simulink model "FCS_MPC_6ph_testbench"  (R2022a)
settings: Solver=ode23t  StartTime=0.0  StopTime=0.1  RelTol=1e-3  AbsTol=1e-3  EnableMultiTasking=on
values from neighbouring files (symbols this model uses):
  f_c = 100000    [Params_testbench.m]
  L_d = 0.0001473    [Params_testbench.m]
  L_q = 0.0001484    [Params_testbench.m]
  L_x = 0.00005566    (= 5.566e-05)    [Params_testbench.m]
  L_y = L_x    (= 5.566e-05)    [Params_testbench.m]
  p = 5    [Params_testbench.m]
  psi_pm = 0.0048    [Params_testbench.m]
  R_ph = 0.1278    [Params_testbench.m]
  u_dc = 36.0    (= 36)    [Params_testbench.m]
libraries: nesl_utility x39, fl_lib x32, hdlsllib x25, ee_lib x12, simulink x2, spsAlphaBetaZerotodq0Lib x1
(part 3 of 4)

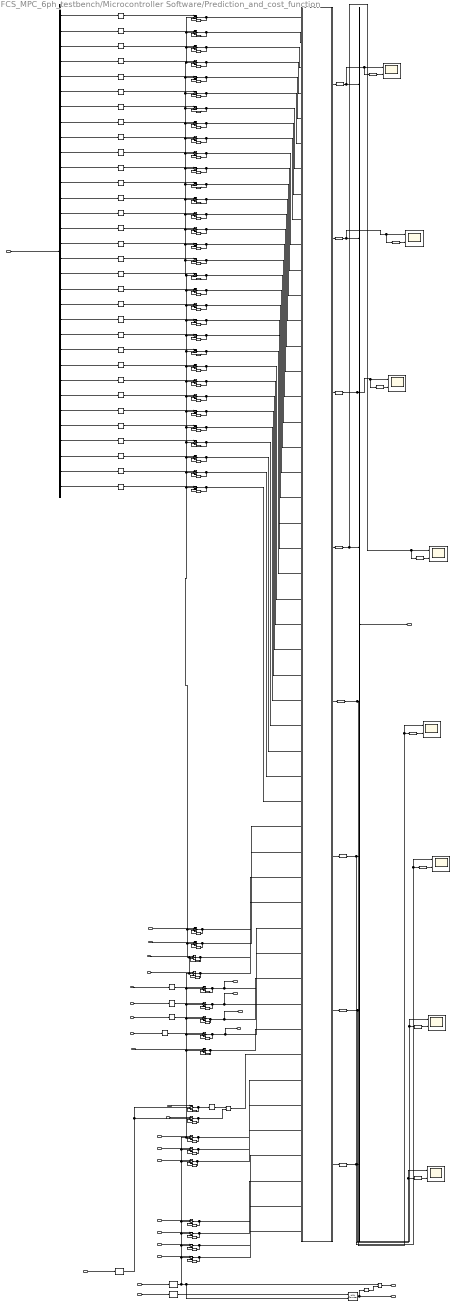
== system FCS_MPC_6ph_testbench/Microcontroller Software/Prediction_and_cost_function ==
  Lq_AXI : Inport
  Ld_AXI : Inport  Port=2
  SampleTime_div_Ld_AXI : Inport  Port=3
  SampleTime_div_Lq_AXI : Inport  Port=4
  SampleTime_div_Lx_AXI : Inport  Port=5
  SampleTime_div_Ly_AXI : Inport  Port=6
  id_k_1 : Inport  Port=7
  iq_k_1 : Inport  Port=8
  ix_k_1 : Inport  Port=9
  iy_k_1 : Inport  Port=10
  Rs_AXI : Inport  Port=11
  omega_m_measured : Inport  Port=12
  pole_pairs_AXI : Inport  Port=13
  psiPM_AXI : Inport  Port=14
  id_ref_AXI : Inport  Port=15
  iq_ref_AXI : Inport  Port=16
  ix_ref_AXI : Inport  Port=17
  iy_ref_AXI : Inport  Port=18
  valid_in : Inport  Port=19
  Reset : Inport  Port=20
  valid_in_ADC : Inport  Port=21
  dqxy_phase_voltage_per_switching_state : Inport  Port=22
  Compare To Constant : hdlsllib/Logic and Bit Operations/Compare To Constant  relop=<=  const=8  OutDataTypeStr=boolean
      settings: SourceProductBaseCode=SL
  Data Type Conversion{1..17,19..38} (37 alike) : DataTypeConversion  OutDataTypeStr=single  RndMeth=Nearest  SaturateOnIntegerOverflow=off
  Data Type Conversion{18,39..52,54} (16 alike) : DataTypeConversion  OutDataTypeStr=fixdt(1,20,9)  SaturateOnIntegerOverflow=off  RndMeth=Floor
  Delay{1..4,8..20,33,104..135} (50 alike) : Delay  DelayLength=1
  Demux : Demux  Outputs=32
  Detect Rise Positive : hdlsllib/Logic and Bit Operations/Detect Rise Positive  vinit=0  OutDataTypeStr=boolean
      settings: SourceProductBaseCode=SL
  Detect Rise Positive1 : hdlsllib/Logic and Bit Operations/Detect Rise Positive  vinit=0  OutDataTypeStr=boolean
      settings: SourceProductBaseCode=SL
  Detect Rise Positive2 : hdlsllib/Logic and Bit Operations/Detect Rise Positive  vinit=0  OutDataTypeStr=boolean
      settings: SourceProductBaseCode=SL
  HDL Counter : hdlsllib/Sources/HDL Counter  CountType=Free running  CountInit=0  CountStep=1  CountMax=25  CountFromType=Initial value  CountFrom=0  CountResetPort=on  CountLoadPort=off  CountEnbPort=on  CountDirPort=off  CountHitOutputPort=off  CountDataType=Signed  CountWordLen=32  CountFracLen=0  CountSampTime=1
  J_fixed_point{,1..7} (8 alike) : Scope  NumInputPorts=2
  Logical Operator : Logic  AllPortsSameDT=off  OutDataTypeStr=boolean
  Mux : Mux  Inputs=8
  Product : Product  Inputs=**
  Subsystem : Subsystem
  Switch_on{1..4,8..10,12..21,59..90} (49 alike) : Switch  Threshold=1  OutDataTypeStr=single  RndMeth=Simplest  SaturateOnIntegerOverflow=off  InputSameDT=off
  Switch_on11 : Switch  Threshold=1  RndMeth=Simplest  SaturateOnIntegerOverflow=off  InputSameDT=off  OutDataTypeStr=Inherit: Same as first input
  done : Outport
  Index : Outport  Port=2
  J : Outport  Port=3
  id_k_1_Prediction : Outport  Port=4
  iq_k_1_Prediction : Outport  Port=5
  ix_k_1_Prediction : Outport  Port=6
  iy_k_1_Prediction : Outport  Port=7
  wires:
  Switch_on12/1 -> Subsystem/41(Rs15), Delay12/1
  Rs_AXI/1 -> Switch_on12/1
  SampleTime_div_Ld_AXI/1 -> Switch_on21/1
  Delay3/1 -> Switch_on3/3
  Delay10/1 -> Switch_on10/3
  iq_ref_AXI/1 -> Switch_on2/1
  Delay17/1 -> Switch_on18/3
  Switch_on10/1 -> Delay10/1, Subsystem/43(Lq15)
  Delay11/1 -> Switch_on11/3
  SampleTime_div_Lq_AXI/1 -> Switch_on20/1
  Ld_AXI/1 -> Switch_on9/1
  psiPM_AXI/1 -> Switch_on8/1
  Delay1/1 -> Switch_on1/3
  id_ref_AXI/1 -> Switch_on3/1
  Product/1 -> Subsystem/42(omega_el15)  "omega_el"
  Delay9/1 -> Switch_on9/3
  Delay20/1 -> Switch_on21/3
  pole_pairs_AXI/1 -> Switch_on4/1
  Switch_on18/1 -> Delay17/1, Subsystem/36(SampleTime_div_Ly15)
  Delay19/1 -> Switch_on20/3
  Delay13/1 -> Switch_on13/3
  Switch_on15/1 -> Delay14/1, ix_k_1_Prediction/1, Subsystem/39(ix_k_16)
  Delay18/1 -> Switch_on19/3
  Switch_on19/1 -> Delay18/1, Subsystem/35(SampleTime_div_Lx15)
  Switch_on20/1 -> Delay19/1, Subsystem/34(SampleTime_div_Lq15)
  Switch_on13/1 -> Delay13/1, iy_k_1_Prediction/1, Subsystem/40(iy_k_16)
  iy_ref_AXI/1 -> Switch_on14/1
  Delay2/1 -> Switch_on2/3
  Delay16/1 -> Switch_on17/3
  Switch_on17/1 -> Delay16/1, id_k_1_Prediction/1, Subsystem/37(id_k_16)
  Delay15/1 -> Switch_on16/3
  Switch_on16/1 -> Delay15/1, iq_k_1_Prediction/1, Subsystem/38(iq_k_16)
  Switch_on11/1 -> Data Type Conversion4/1, Delay11/1
  Delay33/1 -> Switch_on14/3
  SampleTime_div_Lx_AXI/1 -> Switch_on19/1
  Switch_on14/1 -> Delay33/1, Subsystem/49(iy_ref15)
  Delay12/1 -> Switch_on12/3
  valid_in/1 -> Detect Rise Positive/1
  Switch_on3/1 -> Delay3/1, Subsystem/46(id_ref15)
  Switch_on21/1 -> Delay20/1, Subsystem/33(SampleTime_div_Ld15)
  Switch_on2/1 -> Delay2/1, Subsystem/47(iq_ref15)
  Lq_AXI/1 -> Switch_on10/1
  Switch_on1/1 -> Delay1/1, Subsystem/48(ix_ref15)
  Switch_on9/1 -> Delay9/1, Subsystem/44(Ld15)
  SampleTime_div_Ly_AXI/1 -> Switch_on18/1
  Delay14/1 -> Switch_on15/3
  ix_ref_AXI/1 -> Switch_on1/1
  Switch_on8/1 -> Delay8/1, Subsystem/45(psiPM15)
  Delay8/1 -> Switch_on8/3
  id_k_1/1 -> Data Type Conversion7/1
  iq_k_1/1 -> Data Type Conversion8/1
  ix_k_1/1 -> Data Type Conversion9/1
  iy_k_1/1 -> Data Type Conversion10/1
  omega_m_measured/1 -> Switch_on11/1
  Reset/1 -> Detect Rise Positive1/1
  Detect Rise Positive1/1 -> HDL Counter/1  "End_Cycle"
  Compare To Constant/1 -> Logical Operator/2
  HDL Counter/1 -> Index/1, Compare To Constant/1
  valid_in_ADC/1 -> Detect Rise Positive2/1
  Mux/1 -> J/1
  Switch_on61/1 -> Subsystem/30(q_phase_voltage_per_switching_state7), Delay106/1
  Delay106/1 -> Switch_on61/3
  Delay107/1 -> Switch_on62/3
  Switch_on62/1 -> Subsystem/29(d_phase_voltage_per_switching_state7), Delay107/1
  Delay104/1 -> Switch_on59/3
  Switch_on59/1 -> Subsystem/32(y_phase_voltage_per_switching_state7), Delay104/1
  Delay105/1 -> Switch_on60/3
  Switch_on60/1 -> Subsystem/31(x_phase_voltage_per_switching_state7), Delay105/1
  Switch_on65/1 -> Subsystem/26(q_phase_voltage_per_switching_state6), Delay110/1
  Delay110/1 -> Switch_on65/3
  Delay111/1 -> Switch_on66/3
  Switch_on66/1 -> Subsystem/25(d_phase_voltage_per_switching_state6), Delay111/1
  Delay108/1 -> Switch_on63/3
  Switch_on63/1 -> Subsystem/28(y_phase_voltage_per_switching_state6), Delay108/1
  Delay109/1 -> Switch_on64/3
  Switch_on64/1 -> Subsystem/27(x_phase_voltage_per_switching_state6), Delay109/1
  Switch_on69/1 -> Subsystem/22(q_phase_voltage_per_switching_state5), Delay114/1
  Delay114/1 -> Switch_on69/3
  Delay115/1 -> Switch_on70/3
  Switch_on70/1 -> Subsystem/21(d_phase_voltage_per_switching_state5), Delay115/1
  Delay112/1 -> Switch_on67/3
  Switch_on67/1 -> Subsystem/24(y_phase_voltage_per_switching_state5), Delay112/1
  Delay113/1 -> Switch_on68/3
  Switch_on68/1 -> Subsystem/23(x_phase_voltage_per_switching_state5), Delay113/1
  Switch_on73/1 -> Subsystem/18(q_phase_voltage_per_switching_state4), Delay118/1
  Delay118/1 -> Switch_on73/3
  Delay119/1 -> Switch_on74/3
  Switch_on74/1 -> Subsystem/17(d_phase_voltage_per_switching_state4), Delay119/1
  Delay116/1 -> Switch_on71/3
  Switch_on71/1 -> Subsystem/20(y_phase_voltage_per_switching_state4), Delay116/1
  Delay117/1 -> Switch_on72/3
  Switch_on72/1 -> Subsystem/19(x_phase_voltage_per_switching_state4), Delay117/1
  Switch_on77/1 -> Subsystem/14(q_phase_voltage_per_switching_state3), Delay122/1
  Delay122/1 -> Switch_on77/3
  Delay123/1 -> Switch_on78/3
  Switch_on78/1 -> Subsystem/13(d_phase_voltage_per_switching_state3), Delay123/1
  Delay120/1 -> Switch_on75/3
  Switch_on75/1 -> Subsystem/16(y_phase_voltage_per_switching_state3), Delay120/1
  Delay121/1 -> Switch_on76/3
  Switch_on76/1 -> Subsystem/15(x_phase_voltage_per_switching_state3), Delay121/1
  Switch_on81/1 -> Subsystem/10(q_phase_voltage_per_switching_state2), Delay126/1
  Delay126/1 -> Switch_on81/3
  Delay127/1 -> Switch_on82/3
  Switch_on82/1 -> Subsystem/9(d_phase_voltage_per_switching_state2), Delay127/1
  Delay124/1 -> Switch_on79/3
  Switch_on79/1 -> Subsystem/12(y_phase_voltage_per_switching_state2), Delay124/1
  Delay125/1 -> Switch_on80/3
  Switch_on80/1 -> Subsystem/11(x_phase_voltage_per_switching_state2), Delay125/1
  Switch_on85/1 -> Subsystem/6(q_phase_voltage_per_switching_state1), Delay130/1
  Delay130/1 -> Switch_on85/3
  Delay131/1 -> Switch_on86/3
  Switch_on86/1 -> Subsystem/5(d_phase_voltage_per_switching_state1), Delay131/1
  Delay128/1 -> Switch_on83/3
  Switch_on83/1 -> Subsystem/8(y_phase_voltage_per_switching_state1), Delay128/1
  Delay129/1 -> Switch_on84/3
  Switch_on84/1 -> Subsystem/7(x_phase_voltage_per_switching_state1), Delay129/1
  Switch_on89/1 -> Subsystem/2(q_phase_voltage_per_switching_state), Delay134/1
  Delay134/1 -> Switch_on89/3
  Delay135/1 -> Switch_on90/3
  Switch_on90/1 -> Subsystem/1(d_phase_voltage_per_switching_state), Delay135/1
  Delay132/1 -> Switch_on87/3
  Switch_on87/1 -> Subsystem/4(y_phase_voltage_per_switching_state), Delay132/1
  Delay133/1 -> Switch_on88/3
  Switch_on88/1 -> Subsystem/3(x_phase_voltage_per_switching_state), Delay133/1
  Detect Rise Positive/1 -> Logical Operator/1, HDL Counter/2, Switch_on14/2, Switch_on1/2, Switch_on8/2, Switch_on9/2, Switch_on12/2, Switch_on20/2, Switch_on90/2, Switch_on89/2, Switch_on88/2, Switch_on87/2, Switch_on86/2, Switch_on85/2, Switch_on84/2, Switch_on83/2, Switch_on82/2, Switch_on81/2, Switch_on80/2, Switch_on79/2, Switch_on78/2, Switch_on77/2, Switch_on76/2, Switch_on75/2, Switch_on74/2, Switch_on73/2, Switch_on72/2, Switch_on71/2, Switch_on70/2, Switch_on69/2, Switch_on68/2, Switch_on67/2, Switch_on66/2, Switch_on65/2, Switch_on64/2, Switch_on63/2, Switch_on62/2, Switch_on61/2, Switch_on60/2, Switch_on59/2, Switch_on21/2, Switch_on19/2, Switch_on18/2, Switch_on17/2, Switch_on16/2, Switch_on15/2, Switch_on13/2, Switch_on10/2, Switch_on3/2, Switch_on2/2  "End_Cycle"
  Demux/32 -> Data Type Conversion38/1
  Demux/31 -> Data Type Conversion37/1
  Demux/30 -> Data Type Conversion36/1
  Demux/29 -> Data Type Conversion35/1
  Demux/28 -> Data Type Conversion34/1
  Demux/27 -> Data Type Conversion33/1
  Demux/26 -> Data Type Conversion32/1
  Demux/25 -> Data Type Conversion31/1
  Demux/24 -> Data Type Conversion30/1
  Demux/23 -> Data Type Conversion29/1
  Demux/22 -> Data Type Conversion28/1
  Demux/21 -> Data Type Conversion27/1
  Demux/20 -> Data Type Conversion26/1
  Demux/19 -> Data Type Conversion25/1
  Demux/18 -> Data Type Conversion24/1
  Demux/17 -> Data Type Conversion23/1
  Demux/16 -> Data Type Conversion22/1
  Demux/15 -> Data Type Conversion21/1
  Demux/14 -> Data Type Conversion20/1
  Demux/13 -> Data Type Conversion19/1
  Demux/12 -> Data Type Conversion17/1
  Demux/11 -> Data Type Conversion16/1
  Demux/10 -> Data Type Conversion15/1
  Demux/9 -> Data Type Conversion14/1
  Demux/8 -> Data Type Conversion13/1
  Demux/7 -> Data Type Conversion12/1
  Demux/6 -> Data Type Conversion11/1
  Demux/5 -> Data Type Conversion6/1
  Demux/4 -> Data Type Conversion5/1
  Demux/3 -> Data Type Conversion3/1
  Demux/2 -> Data Type Conversion2/1
  Demux/1 -> Data Type Conversion1/1
  Logical Operator/1 -> done/1
  dqxy_phase_voltage_per_switching_state/1 -> Demux/1
  Data Type Conversion10/1 -> Switch_on13/1
  Data Type Conversion9/1 -> Switch_on15/1
  Data Type Conversion8/1 -> Switch_on16/1
  Data Type Conversion7/1 -> Switch_on17/1
  Data Type Conversion4/1 -> Product/1
  Data Type Conversion38/1 -> Switch_on59/1
  Data Type Conversion37/1 -> Switch_on60/1
  Data Type Conversion36/1 -> Switch_on61/1
  Data Type Conversion35/1 -> Switch_on62/1
  Data Type Conversion34/1 -> Switch_on63/1
  Data Type Conversion33/1 -> Switch_on64/1
  Data Type Conversion32/1 -> Switch_on65/1
  Data Type Conversion31/1 -> Switch_on66/1
  Data Type Conversion30/1 -> Switch_on67/1
  Data Type Conversion29/1 -> Switch_on68/1
  Data Type Conversion28/1 -> Switch_on69/1
  Data Type Conversion27/1 -> Switch_on70/1
  Data Type Conversion26/1 -> Switch_on71/1
  Data Type Conversion25/1 -> Switch_on72/1
  Data Type Conversion24/1 -> Switch_on73/1
  Data Type Conversion23/1 -> Switch_on74/1
  Data Type Conversion22/1 -> Switch_on75/1
  Data Type Conversion21/1 -> Switch_on76/1
  Data Type Conversion20/1 -> Switch_on77/1
  Data Type Conversion19/1 -> Switch_on78/1
  Data Type Conversion17/1 -> Switch_on79/1
  Data Type Conversion16/1 -> Switch_on80/1
  Data Type Conversion15/1 -> Switch_on81/1
  Data Type Conversion14/1 -> Switch_on82/1
  Data Type Conversion13/1 -> Switch_on83/1
  Data Type Conversion12/1 -> Switch_on84/1
  Data Type Conversion11/1 -> Switch_on85/1
  Data Type Conversion6/1 -> Switch_on86/1
  Data Type Conversion5/1 -> Switch_on87/1
  Data Type Conversion3/1 -> Switch_on88/1
  Data Type Conversion2/1 -> Switch_on89/1
  Data Type Conversion1/1 -> Switch_on90/1
  Detect Rise Positive2/1 -> Switch_on4/2, Switch_on11/2  "End_Cycle"
  Switch_on4/1 -> Product/2, Delay4/1
  Delay4/1 -> Switch_on4/3
  Data Type Conversion18/1 -> J_fixed_point/2  "fc"
  Data Type Conversion39/1 -> J_fixed_point1/2  "fc"
  Data Type Conversion40/1 -> J_fixed_point2/2  "fc"
  Data Type Conversion41/1 -> J_fixed_point3/2  "fc"
  Data Type Conversion42/1 -> J_fixed_point4/2  "fc"
  Data Type Conversion43/1 -> J_fixed_point5/2  "fc"
  Data Type Conversion44/1 -> J_fixed_point6/2  "fc"
  Data Type Conversion45/1 -> J_fixed_point7/2  "fc"
  Subsystem/8(J7) -> Data Type Conversion52/1  "fc"
  Subsystem/7(J6) -> Data Type Conversion51/1  "fc"
  Subsystem/6(J5) -> Data Type Conversion50/1  "fc"
  Subsystem/5(J4) -> Data Type Conversion49/1  "fc"
  Subsystem/4(J3) -> Data Type Conversion48/1  "fc"
  Subsystem/3(J2) -> Data Type Conversion47/1  "fc"
  Subsystem/2(J1) -> Data Type Conversion46/1  "fc"
  Subsystem/1(J) -> Data Type Conversion54/1  "fc"
  Data Type Conversion54/1 -> Data Type Conversion18/1, J_fixed_point/1, Mux/1  "fc"
  Data Type Conversion46/1 -> Data Type Conversion39/1, J_fixed_point1/1, Mux/2  "fc"
  Data Type Conversion47/1 -> Data Type Conversion40/1, J_fixed_point2/1, Mux/3  "fc"
  Data Type Conversion48/1 -> Data Type Conversion41/1, J_fixed_point3/1, Mux/4  "fc"
  Data Type Conversion49/1 -> J_fixed_point4/1, Data Type Conversion42/1, Mux/5  "fc"
  Data Type Conversion50/1 -> J_fixed_point5/1, Data Type Conversion43/1, Mux/6  "fc"
  Data Type Conversion51/1 -> J_fixed_point6/1, Data Type Conversion44/1, Mux/7  "fc"
  Data Type Conversion52/1 -> J_fixed_point7/1, Data Type Conversion45/1, Mux/8  "fc"

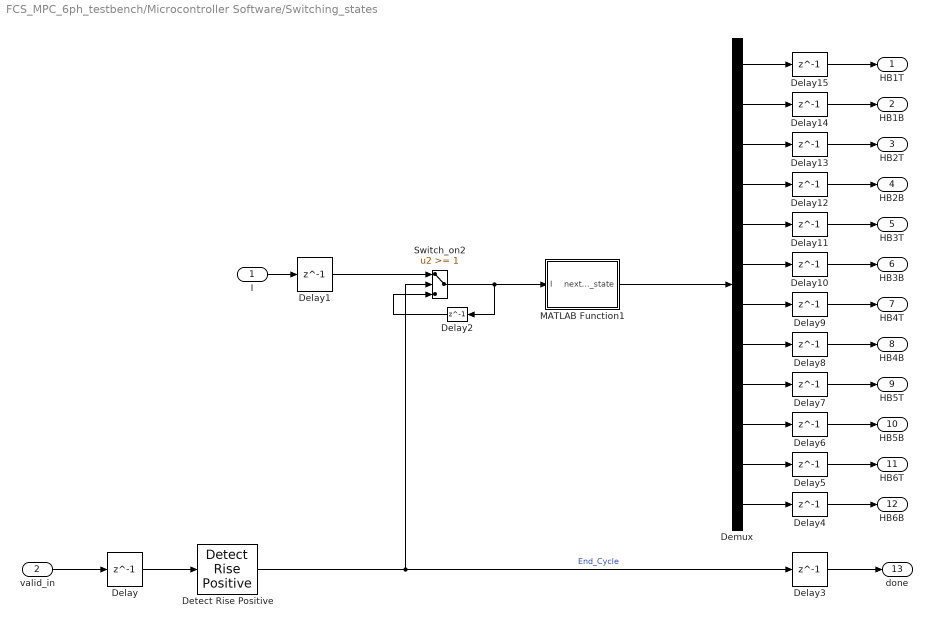
== system FCS_MPC_6ph_testbench/Microcontroller Software/Switching_states ==
  I : Inport
  valid_in : Inport  Port=2
  Delay{,1..15} (16 alike) : Delay  DelayLength=1
  Demux : Demux  Outputs=12
  Detect Rise Positive : hdlsllib/Logic and Bit Operations/Detect Rise Positive  vinit=0  OutDataTypeStr=boolean
      settings: SourceProductBaseCode=SL
  MATLAB Function1 : MATLAB Function  TreatAsAtomicUnit=on
  Switch_on2 : Switch  Threshold=1  OutDataTypeStr=Inherit: Inherit via back propagation  RndMeth=Simplest  SaturateOnIntegerOverflow=off  InputSameDT=off
  HB1T : Outport
  HB1B : Outport  Port=2
  HB2T : Outport  Port=3
  HB2B : Outport  Port=4
  HB3T : Outport  Port=5
  HB3B : Outport  Port=6
  HB4T : Outport  Port=7
  HB4B : Outport  Port=8
  HB5T : Outport  Port=9
  HB5B : Outport  Port=10
  HB6T : Outport  Port=11
  HB6B : Outport  Port=12
  done : Outport  Port=13
  wires:
  Demux/4 -> Delay12/1
  I/1 -> Delay1/1
  Demux/6 -> Delay10/1
  Demux/12 -> Delay4/1
  Demux/8 -> Delay8/1
  valid_in/1 -> Delay/1
  Demux/7 -> Delay9/1
  Demux/2 -> Delay14/1
  Detect Rise Positive/1 -> Delay3/1, Switch_on2/2  "End_Cycle"
  Demux/5 -> Delay11/1
  Delay2/1 -> Switch_on2/3
  Demux/1 -> Delay15/1
  Demux/9 -> Delay7/1
  Demux/10 -> Delay6/1
  MATLAB Function1/1(next_switching_state) -> Demux/1
  Demux/3 -> Delay13/1
  Delay/1 -> Detect Rise Positive/1
  Delay1/1 -> Switch_on2/1
  Delay3/1 -> done/1
  Delay4/1 -> HB6B/1
  Demux/11 -> Delay5/1
  Delay5/1 -> HB6T/1
  Delay6/1 -> HB5B/1
  Delay7/1 -> HB5T/1
  Delay8/1 -> HB4B/1
  Delay9/1 -> HB4T/1
  Delay10/1 -> HB3B/1
  Delay11/1 -> HB3T/1
  Delay12/1 -> HB2B/1
  Delay13/1 -> HB2T/1
  Delay14/1 -> HB1B/1
  Delay15/1 -> HB1T/1
  Switch_on2/1 -> MATLAB Function1/1(I), Delay2/1

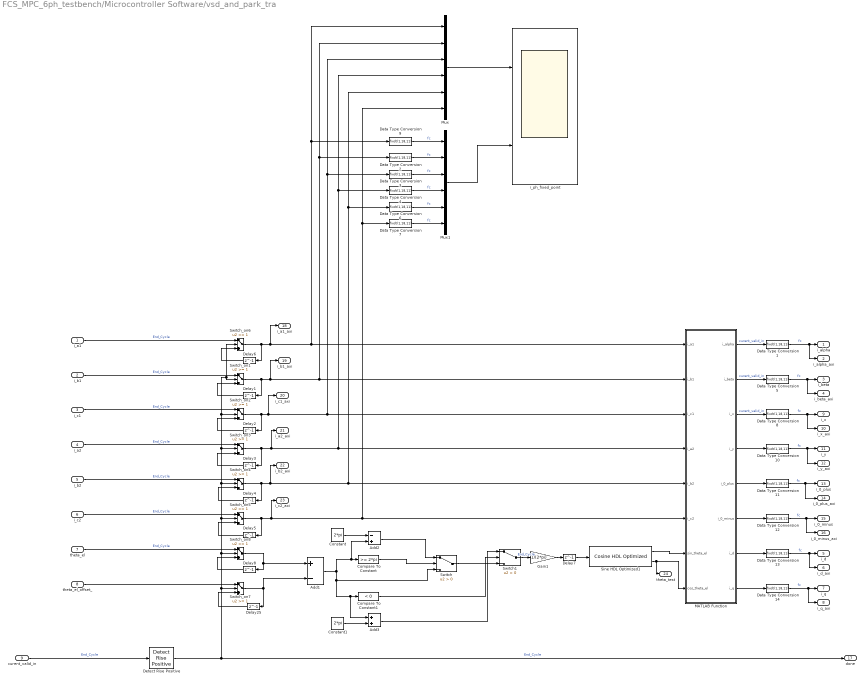
== system FCS_MPC_6ph_testbench/Microcontroller Software/vsd_and_park_tra ==
  i_a1 : Inport
  i_b1 : Inport  Port=2
  i_c1 : Inport  Port=3
  i_a2 : Inport  Port=4
  i_b2 : Inport  Port=5
  i_c2 : Inport  Port=6
  theta_el : Inport  Port=7
  theta_el_offset_ : Inport  Port=8
  curent_valid_in : Inport  Port=9
  Add1 : Sum  Inputs=+-  RndMeth=Simplest  OutDataTypeStr=Inherit: Same as first input
  Add2 : Sum  Inputs=-+  RndMeth=Simplest  OutDataTypeStr=Inherit: Same as first input
  Add3 : Sum  RndMeth=Simplest  OutDataTypeStr=Inherit: Same as first input
  Compare To Constant : hdlsllib/Logic and Bit Operations/Compare To Constant  relop=>=  const=2*pi  OutDataTypeStr=boolean
      settings: SourceProductBaseCode=SL
  Compare To Constant1 : hdlsllib/Logic and Bit Operations/Compare To Constant  relop=<  const=0  OutDataTypeStr=boolean
      settings: SourceProductBaseCode=SL
  Constant : Constant  Value=2*pi  OutDataTypeStr=fixdt(1,24,20)  SampleTime=1.0000e-08
  Constant1 : Constant  Value=2*pi  OutDataTypeStr=fixdt(1,24,20)  SampleTime=1.0000e-08
  Data Type Conversion{1..14} (14 alike) : DataTypeConversion  OutDataTypeStr=fixdt(1,18,11)  SaturateOnIntegerOverflow=off  RndMeth=Floor
  Delay{1..8,25} (9 alike) : Delay  DelayLength=1
  Detect Rise Positive : hdlsllib/Logic and Bit Operations/Detect Rise Positive  vinit=0  OutDataTypeStr=boolean
      settings: SourceProductBaseCode=SL
  Gain1 : Gain  Gain=1/(2*pi)  OutDataTypeStr=Inherit: Same as input  ParamDataTypeStr=Inherit: Same as input
  MATLAB Function : MATLAB Function  TreatAsAtomicUnit=on  SystemSampleTime=1/100000000
  Mux : Mux  Inputs=6
  Mux1 : Mux  Inputs=6
  Sine HDL Optimized1 : hdlsllib/Lookup Tables/Cosine HDL Optimized  OutputFormula=sin(2*pi*u) and cos(2*pi*u)  NumDataPoints=512  TableDataTypeStr=fixdt(1,15,14)  SimulateLUTROMDelay=off
      settings: SourceProductBaseCode=SL
  Switch : Switch  Criteria=u2 > Threshold  RndMeth=Simplest  SaturateOnIntegerOverflow=off  InputSameDT=off  OutDataTypeStr=Inherit: Same as first input
  Switch1 : Switch  Criteria=u2 > Threshold  RndMeth=Simplest  SaturateOnIntegerOverflow=off  InputSameDT=off  OutDataTypeStr=Inherit: Same as first input
  Switch_on{1..8} (8 alike) : Switch  Threshold=1  RndMeth=Simplest  SaturateOnIntegerOverflow=off  InputSameDT=off  OutDataTypeStr=Inherit: Same as first input
  i_ph_fixed_point : Scope  NumInputPorts=2
  i_alpha : Outport
  i_alpha_axi : Outport  Port=2
  i_beta : Outport  Port=3
  i_beta_axi : Outport  Port=4
  i_d : Outport  Port=5
  i_d_axi : Outport  Port=6
  i_q : Outport  Port=7
  i_q_axi : Outport  Port=8
  i_x : Outport  Port=9
  i_x_axi : Outport  Port=10
  i_y : Outport  Port=11
  i_y_axi : Outport  Port=12
  i_0_plus : Outport  Port=13
  i_0_plus_axi : Outport  Port=14
  i_0_minus : Outport  Port=15
  i_0_minus_axi : Outport  Port=16
  done : Outport  Port=17
  i_a1_axi : Outport  Port=18
  i_b1_axi : Outport  Port=19
  i_c1_axi : Outport  Port=20
  i_a2_axi : Outport  Port=21
  i_b2_axi : Outport  Port=22
  i_c2_axi : Outport  Port=23
  theta_test : Outport  Port=24
  wires:
  i_c2/1 -> Switch_on5/1  "End_Cycle"
  Delay8/1 -> Switch_on8/3
  Detect Rise Positive/1 -> done/1, Switch_on7/2, Switch_on6/2, Switch_on1/2, Switch_on2/2, Switch_on3/2, Switch_on4/2, Switch_on5/2, Switch_on8/2  "End_Cycle"
  Delay4/1 -> Switch_on4/3
  Switch_on2/1 -> Delay2/1, i_c1_axi/1, Mux/3, Data Type Conversion3/1, MATLAB Function/3(i_c1)
  Delay1/1 -> Switch_on1/3
  Switch_on1/1 -> Delay1/1, i_b1_axi/1, Mux/2, Data Type Conversion2/1, MATLAB Function/2(i_b1)
  Switch_on6/1 -> i_a1_axi/1, Mux/1, Data Type Conversion9/1, MATLAB Function/1(i_a1), Delay6/1
  Switch_on4/1 -> Delay4/1, i_b2_axi/1, Mux/5, Data Type Conversion6/1, MATLAB Function/5(i_b2)
  curent_valid_in/1 -> Detect Rise Positive/1  "End_Cycle"
  Switch/1 -> Switch1/3
  Switch_on3/1 -> i_a2_axi/1, Mux/4, Data Type Conversion4/1, MATLAB Function/4(i_a2), Delay3/1
  Delay6/1 -> Switch_on6/3
  Constant/1 -> Add2/1
  Add1/1 -> Switch/3, Compare To Constant1/1, Add3/1, Compare To Constant/1, Add2/2
  Delay2/1 -> Switch_on2/3
  Constant1/1 -> Add3/2
  theta_el/1 -> Switch_on8/1  "End_Cycle"
  Delay3/1 -> Switch_on3/3
  i_a1/1 -> Switch_on6/1  "End_Cycle"
  i_b2/1 -> Switch_on4/1  "End_Cycle"
  Add2/1 -> Switch/1
  i_a2/1 -> Switch_on3/1  "End_Cycle"
  i_b1/1 -> Switch_on1/1  "End_Cycle"
  Delay5/1 -> Switch_on5/3
  Add3/1 -> Switch1/1
  i_c1/1 -> Switch_on2/1  "End_Cycle"
  MATLAB Function/1(i_alpha) -> Data Type Conversion1/1  "curent_valid_in"
  MATLAB Function/2(i_beta) -> Data Type Conversion5/1  "curent_valid_in"
  MATLAB Function/3(i_x) -> Data Type Conversion8/1  "curent_valid_in"
  Compare To Constant/1 -> Switch/2
  Compare To Constant1/1 -> Switch1/2
  Delay25/1 -> Switch_on7/3
  theta_el_offset_/1 -> Switch_on7/1
  MATLAB Function/8(i_q) -> Data Type Conversion14/1
  MATLAB Function/7(i_d) -> Data Type Conversion13/1
  MATLAB Function/6(i_0_minus) -> Data Type Conversion12/1
  MATLAB Function/5(i_0_plus) -> Data Type Conversion11/1
  MATLAB Function/4(i_y) -> Data Type Conversion10/1
  Switch_on5/1 -> Delay5/1, i_c2_axi/1, Data Type Conversion7/1, Mux/6, MATLAB Function/6(i_c2)
  Mux/1 -> i_ph_fixed_point/1
  Mux1/1 -> i_ph_fixed_point/2
  Data Type Conversion9/1 -> Mux1/1  "fc"
  Data Type Conversion2/1 -> Mux1/2  "fc"
  Data Type Conversion3/1 -> Mux1/3  "fc"
  Data Type Conversion4/1 -> Mux1/4  "fc"
  Data Type Conversion6/1 -> Mux1/5  "fc"
  Data Type Conversion7/1 -> Mux1/6  "fc"
  Data Type Conversion1/1 -> i_alpha_axi/1, i_alpha/1  "fc"
  Data Type Conversion5/1 -> i_beta_axi/1, i_beta/1  "fc"
  Data Type Conversion8/1 -> i_x_axi/1, i_x/1  "fc"
  Data Type Conversion10/1 -> i_y_axi/1, i_y/1  "fc"
  Data Type Conversion11/1 -> i_0_plus_axi/1, i_0_plus/1  "fc"
  Data Type Conversion12/1 -> i_0_minus_axi/1, i_0_minus/1  "fc"
  Data Type Conversion13/1 -> i_d_axi/1, i_d/1  "fc"
  Data Type Conversion14/1 -> i_q_axi/1, i_q/1  "fc"
  Sine HDL Optimized1/1 -> MATLAB Function/7(sin_theta_el)
  Switch_on8/1 -> Add1/1, Delay8/1
  Switch_on7/1 -> Add1/2, Delay25/1
  Delay7/1 -> Sine HDL Optimized1/1
  Gain1/1 -> Delay7/1
  Switch1/1 -> Gain1/1  "End_Cycle"
  Sine HDL Optimized1/2 -> theta_test/1, MATLAB Function/8(cos_theta_el)

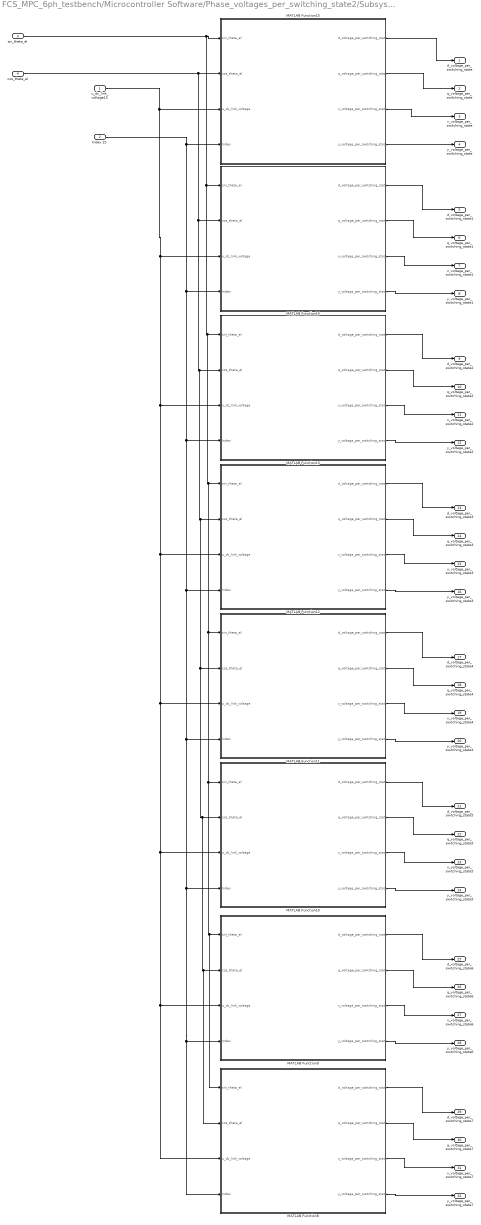
== system FCS_MPC_6ph_testbench/Microcontroller Software/Phase_voltages_per_switching_state2/Subsystem ==
  u_dc_link_voltage15 : Inport
  Index 15 : Inport  Port=2
  sin_theta_el : Inport  Port=3
  cos_theta_el : Inport  Port=4
  MATLAB Function10 : MATLAB Function  TreatAsAtomicUnit=on  SystemSampleTime=1/100000000
  MATLAB Function11 : MATLAB Function  TreatAsAtomicUnit=on  SystemSampleTime=1/100000000
  MATLAB Function12 : MATLAB Function  TreatAsAtomicUnit=on  SystemSampleTime=1/100000000
  MATLAB Function13 : MATLAB Function  TreatAsAtomicUnit=on  SystemSampleTime=1/100000000
  MATLAB Function14 : MATLAB Function  TreatAsAtomicUnit=on  SystemSampleTime=1/100000000
  MATLAB Function15 : MATLAB Function  TreatAsAtomicUnit=on  SystemSampleTime=1/100000000
  MATLAB Function8 : MATLAB Function  TreatAsAtomicUnit=on  SystemSampleTime=1/100000000
  MATLAB Function9 : MATLAB Function  TreatAsAtomicUnit=on  SystemSampleTime=1/100000000
  d_voltage_per_switching_state : Outport
  q_voltage_per_switching_state : Outport  Port=2
  x_voltage_per_switching_state : Outport  Port=3
  y_voltage_per_switching_state : Outport  Port=4
  d_voltage_per_switching_state1 : Outport  Port=5
  q_voltage_per_switching_state1 : Outport  Port=6
  x_voltage_per_switching_state1 : Outport  Port=7
  y_voltage_per_switching_state1 : Outport  Port=8
  d_voltage_per_switching_state2 : Outport  Port=9
  q_voltage_per_switching_state2 : Outport  Port=10
  x_voltage_per_switching_state2 : Outport  Port=11
  y_voltage_per_switching_state2 : Outport  Port=12
  d_voltage_per_switching_state3 : Outport  Port=13
  q_voltage_per_switching_state3 : Outport  Port=14
  x_voltage_per_switching_state3 : Outport  Port=15
  y_voltage_per_switching_state3 : Outport  Port=16
  d_voltage_per_switching_state4 : Outport  Port=17
  q_voltage_per_switching_state4 : Outport  Port=18
  x_voltage_per_switching_state4 : Outport  Port=19
  y_voltage_per_switching_state4 : Outport  Port=20
  d_voltage_per_switching_state5 : Outport  Port=21
  q_voltage_per_switching_state5 : Outport  Port=22
  x_voltage_per_switching_state5 : Outport  Port=23
  y_voltage_per_switching_state5 : Outport  Port=24
  d_voltage_per_switching_state6 : Outport  Port=25
  q_voltage_per_switching_state6 : Outport  Port=26
  x_voltage_per_switching_state6 : Outport  Port=27
  y_voltage_per_switching_state6 : Outport  Port=28
  d_voltage_per_switching_state7 : Outport  Port=29
  q_voltage_per_switching_state7 : Outport  Port=30
  x_voltage_per_switching_state7 : Outport  Port=31
  y_voltage_per_switching_state7 : Outport  Port=32
  wires:
  MATLAB Function11/4(y_voltage_per_switching_state) -> y_voltage_per_switching_state4/1
  MATLAB Function10/3(x_voltage_per_switching_state) -> x_voltage_per_switching_state5/1
  MATLAB Function8/1(d_voltage_per_switching_state) -> d_voltage_per_switching_state7/1
  MATLAB Function8/2(q_voltage_per_switching_state) -> q_voltage_per_switching_state7/1
  MATLAB Function11/1(d_voltage_per_switching_state) -> d_voltage_per_switching_state4/1
  MATLAB Function12/3(x_voltage_per_switching_state) -> x_voltage_per_switching_state3/1
  MATLAB Function15/2(q_voltage_per_switching_state) -> q_voltage_per_switching_state/1
  MATLAB Function8/3(x_voltage_per_switching_state) -> x_voltage_per_switching_state7/1
  MATLAB Function11/3(x_voltage_per_switching_state) -> x_voltage_per_switching_state4/1
  MATLAB Function10/4(y_voltage_per_switching_state) -> y_voltage_per_switching_state5/1
  MATLAB Function11/2(q_voltage_per_switching_state) -> q_voltage_per_switching_state4/1
  MATLAB Function12/1(d_voltage_per_switching_state) -> d_voltage_per_switching_state3/1
  MATLAB Function12/4(y_voltage_per_switching_state) -> y_voltage_per_switching_state3/1
  MATLAB Function13/2(q_voltage_per_switching_state) -> q_voltage_per_switching_state2/1
  MATLAB Function10/1(d_voltage_per_switching_state) -> d_voltage_per_switching_state5/1
  MATLAB Function10/2(q_voltage_per_switching_state) -> q_voltage_per_switching_state5/1
  MATLAB Function13/4(y_voltage_per_switching_state) -> y_voltage_per_switching_state2/1
  MATLAB Function8/4(y_voltage_per_switching_state) -> y_voltage_per_switching_state7/1
  MATLAB Function13/1(d_voltage_per_switching_state) -> d_voltage_per_switching_state2/1
  MATLAB Function13/3(x_voltage_per_switching_state) -> x_voltage_per_switching_state2/1
  MATLAB Function12/2(q_voltage_per_switching_state) -> q_voltage_per_switching_state3/1
  MATLAB Function15/1(d_voltage_per_switching_state) -> d_voltage_per_switching_state/1
  MATLAB Function15/4(y_voltage_per_switching_state) -> y_voltage_per_switching_state/1
  MATLAB Function15/3(x_voltage_per_switching_state) -> x_voltage_per_switching_state/1
  u_dc_link_voltage15/1 -> MATLAB Function8/3(u_dc_link_voltage), MATLAB Function9/3(u_dc_link_voltage), MATLAB Function10/3(u_dc_link_voltage), MATLAB Function11/3(u_dc_link_voltage), MATLAB Function12/3(u_dc_link_voltage), MATLAB Function13/3(u_dc_link_voltage), MATLAB Function14/3(u_dc_link_voltage), MATLAB Function15/3(u_dc_link_voltage)
  MATLAB Function14/4(y_voltage_per_switching_state) -> y_voltage_per_switching_state1/1
  MATLAB Function14/3(x_voltage_per_switching_state) -> x_voltage_per_switching_state1/1
  MATLAB Function14/1(d_voltage_per_switching_state) -> d_voltage_per_switching_state1/1
  MATLAB Function14/2(q_voltage_per_switching_state) -> q_voltage_per_switching_state1/1
  Index 15/1 -> MATLAB Function15/4(Index), MATLAB Function10/4(Index), MATLAB Function8/4(Index), MATLAB Function9/4(Index), MATLAB Function11/4(Index), MATLAB Function12/4(Index), MATLAB Function13/4(Index), MATLAB Function14/4(Index)
  MATLAB Function9/3(x_voltage_per_switching_state) -> x_voltage_per_switching_state6/1
  MATLAB Function9/2(q_voltage_per_switching_state) -> q_voltage_per_switching_state6/1
  MATLAB Function9/1(d_voltage_per_switching_state) -> d_voltage_per_switching_state6/1
  MATLAB Function9/4(y_voltage_per_switching_state) -> y_voltage_per_switching_state6/1
  sin_theta_el/1 -> MATLAB Function14/1(sin_theta_el), MATLAB Function8/1(sin_theta_el), MATLAB Function9/1(sin_theta_el), MATLAB Function10/1(sin_theta_el), MATLAB Function11/1(sin_theta_el), MATLAB Function12/1(sin_theta_el), MATLAB Function13/1(sin_theta_el), MATLAB Function15/1(sin_theta_el)
  cos_theta_el/1 -> MATLAB Function15/2(cos_theta_el), MATLAB Function8/2(cos_theta_el), MATLAB Function9/2(cos_theta_el), MATLAB Function10/2(cos_theta_el), MATLAB Function11/2(cos_theta_el), MATLAB Function12/2(cos_theta_el), MATLAB Function13/2(cos_theta_el), MATLAB Function14/2(cos_theta_el)

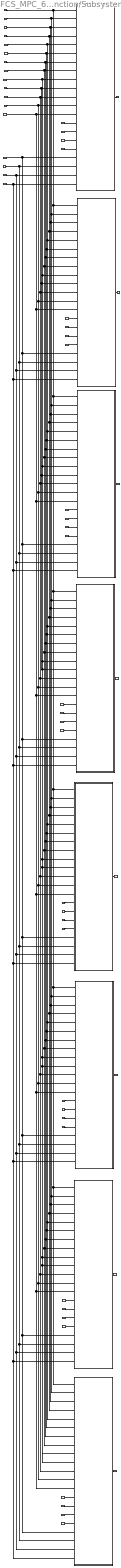
== system FCS_MPC_6ph_testbench/Microcontroller Software/Prediction_and_cost_function/Subsystem ==
  d_phase_voltage_per_switching_state : Inport
  q_phase_voltage_per_switching_state : Inport  Port=2
  x_phase_voltage_per_switching_state : Inport  Port=3
  y_phase_voltage_per_switching_state : Inport  Port=4
  d_phase_voltage_per_switching_state1 : Inport  Port=5
  q_phase_voltage_per_switching_state1 : Inport  Port=6
  x_phase_voltage_per_switching_state1 : Inport  Port=7
  y_phase_voltage_per_switching_state1 : Inport  Port=8
  d_phase_voltage_per_switching_state2 : Inport  Port=9
  q_phase_voltage_per_switching_state2 : Inport  Port=10
  x_phase_voltage_per_switching_state2 : Inport  Port=11
  y_phase_voltage_per_switching_state2 : Inport  Port=12
  d_phase_voltage_per_switching_state3 : Inport  Port=13
  q_phase_voltage_per_switching_state3 : Inport  Port=14
  x_phase_voltage_per_switching_state3 : Inport  Port=15
  y_phase_voltage_per_switching_state3 : Inport  Port=16
  d_phase_voltage_per_switching_state4 : Inport  Port=17
  q_phase_voltage_per_switching_state4 : Inport  Port=18
  x_phase_voltage_per_switching_state4 : Inport  Port=19
  y_phase_voltage_per_switching_state4 : Inport  Port=20
  d_phase_voltage_per_switching_state5 : Inport  Port=21
  q_phase_voltage_per_switching_state5 : Inport  Port=22
  x_phase_voltage_per_switching_state5 : Inport  Port=23
  y_phase_voltage_per_switching_state5 : Inport  Port=24
  d_phase_voltage_per_switching_state6 : Inport  Port=25
  q_phase_voltage_per_switching_state6 : Inport  Port=26
  x_phase_voltage_per_switching_state6 : Inport  Port=27
  y_phase_voltage_per_switching_state6 : Inport  Port=28
  d_phase_voltage_per_switching_state7 : Inport  Port=29
  q_phase_voltage_per_switching_state7 : Inport  Port=30
  x_phase_voltage_per_switching_state7 : Inport  Port=31
  y_phase_voltage_per_switching_state7 : Inport  Port=32
  SampleTime_div_Ld15 : Inport  Port=33
  SampleTime_div_Lq15 : Inport  Port=34
  SampleTime_div_Lx15 : Inport  Port=35
  SampleTime_div_Ly15 : Inport  Port=36
  id_k_16 : Inport  Port=37
  iq_k_16 : Inport  Port=38
  ix_k_16 : Inport  Port=39
  iy_k_16 : Inport  Port=40
  Rs15 : Inport  Port=41
  omega_el15 : Inport  Port=42
  Lq15 : Inport  Port=43
  Ld15 : Inport  Port=44
  psiPM15 : Inport  Port=45
  id_ref15 : Inport  Port=46
  iq_ref15 : Inport  Port=47
  ix_ref15 : Inport  Port=48
  iy_ref15 : Inport  Port=49
  MATLAB Function10 : MATLAB Function  TreatAsAtomicUnit=on  SystemSampleTime=1/100000000
  MATLAB Function11 : MATLAB Function  TreatAsAtomicUnit=on  SystemSampleTime=1/100000000
  MATLAB Function12 : MATLAB Function  TreatAsAtomicUnit=on  SystemSampleTime=1/100000000
  MATLAB Function13 : MATLAB Function  TreatAsAtomicUnit=on  SystemSampleTime=1/100000000
  MATLAB Function14 : MATLAB Function  TreatAsAtomicUnit=on  SystemSampleTime=1/100000000
  MATLAB Function15 : MATLAB Function  TreatAsAtomicUnit=on  SystemSampleTime=1/100000000
  MATLAB Function8 : MATLAB Function  TreatAsAtomicUnit=on  SystemSampleTime=1/100000000
  MATLAB Function9 : MATLAB Function  TreatAsAtomicUnit=on  SystemSampleTime=1/100000000
  J : Outport
  J1 : Outport  Port=2
  J2 : Outport  Port=3
  J3 : Outport  Port=4
  J4 : Outport  Port=5
  J5 : Outport  Port=6
  J6 : Outport  Port=7
  J7 : Outport  Port=8
  wires:
  q_phase_voltage_per_switching_state1/1 -> MATLAB Function14/15(q_phase_voltage_per_switching_state)
  SampleTime_div_Ld15/1 -> MATLAB Function8/1(SampleTime_div_Ld), MATLAB Function9/1(SampleTime_div_Ld), MATLAB Function10/1(SampleTime_div_Ld), MATLAB Function11/1(SampleTime_div_Ld), MATLAB Function12/1(SampleTime_div_Ld), MATLAB Function13/1(SampleTime_div_Ld), MATLAB Function14/1(SampleTime_div_Ld), MATLAB Function15/1(SampleTime_div_Ld)
  Rs15/1 -> MATLAB Function8/9(Rs), MATLAB Function9/9(Rs), MATLAB Function10/9(Rs), MATLAB Function11/9(Rs), MATLAB Function12/9(Rs), MATLAB Function13/9(Rs), MATLAB Function14/9(Rs), MATLAB Function15/9(Rs)
  y_phase_voltage_per_switching_state/1 -> MATLAB Function15/17(y_phase_voltage_per_switching_state)
  Lq15/1 -> MATLAB Function8/11(Lq), MATLAB Function9/11(Lq), MATLAB Function10/11(Lq), MATLAB Function11/11(Lq), MATLAB Function12/11(Lq), MATLAB Function13/11(Lq), MATLAB Function14/11(Lq), MATLAB Function15/11(Lq)
  MATLAB Function11/1(J) -> J4/1
  y_phase_voltage_per_switching_state2/1 -> MATLAB Function13/17(y_phase_voltage_per_switching_state)
  d_phase_voltage_per_switching_state1/1 -> MATLAB Function14/14(d_phase_voltage_per_switching_state)
  x_phase_voltage_per_switching_state1/1 -> MATLAB Function14/16(x_phase_voltage_per_switching_state)
  y_phase_voltage_per_switching_state7/1 -> MATLAB Function8/17(y_phase_voltage_per_switching_state)
  iy_ref15/1 -> MATLAB Function8/21(iy_ref), MATLAB Function9/21(iy_ref), MATLAB Function10/21(iy_ref), MATLAB Function11/21(iy_ref), MATLAB Function12/21(iy_ref), MATLAB Function13/21(iy_ref), MATLAB Function14/21(iy_ref), MATLAB Function15/21(iy_ref)
  omega_el15/1 -> MATLAB Function8/10(omega_el), MATLAB Function9/10(omega_el), MATLAB Function10/10(omega_el), MATLAB Function11/10(omega_el), MATLAB Function12/10(omega_el), MATLAB Function13/10(omega_el), MATLAB Function14/10(omega_el), MATLAB Function15/10(omega_el)
  psiPM15/1 -> MATLAB Function8/13(psiPM), MATLAB Function9/13(psiPM), MATLAB Function10/13(psiPM), MATLAB Function11/13(psiPM), MATLAB Function12/13(psiPM), MATLAB Function13/13(psiPM), MATLAB Function14/13(psiPM), MATLAB Function15/13(psiPM)
  d_phase_voltage_per_switching_state3/1 -> MATLAB Function12/14(d_phase_voltage_per_switching_state)
  d_phase_voltage_per_switching_state6/1 -> MATLAB Function9/14(d_phase_voltage_per_switching_state)
  d_phase_voltage_per_switching_state/1 -> MATLAB Function15/14(d_phase_voltage_per_switching_state)
  x_phase_voltage_per_switching_state3/1 -> MATLAB Function12/16(x_phase_voltage_per_switching_state)
  d_phase_voltage_per_switching_state2/1 -> MATLAB Function13/14(d_phase_voltage_per_switching_state)
  x_phase_voltage_per_switching_state4/1 -> MATLAB Function11/16(x_phase_voltage_per_switching_state)
  y_phase_voltage_per_switching_state1/1 -> MATLAB Function14/17(y_phase_voltage_per_switching_state)
  MATLAB Function14/1(J) -> J1/1
  MATLAB Function8/1(J) -> J7/1
  q_phase_voltage_per_switching_state2/1 -> MATLAB Function13/15(q_phase_voltage_per_switching_state)
  x_phase_voltage_per_switching_state2/1 -> MATLAB Function13/16(x_phase_voltage_per_switching_state)
  MATLAB Function13/1(J) -> J2/1
  y_phase_voltage_per_switching_state4/1 -> MATLAB Function11/17(y_phase_voltage_per_switching_state)
  x_phase_voltage_per_switching_state/1 -> MATLAB Function15/16(x_phase_voltage_per_switching_state)
  q_phase_voltage_per_switching_state5/1 -> MATLAB Function10/15(q_phase_voltage_per_switching_state)
  d_phase_voltage_per_switching_state7/1 -> MATLAB Function8/14(d_phase_voltage_per_switching_state)
  d_phase_voltage_per_switching_state4/1 -> MATLAB Function11/14(d_phase_voltage_per_switching_state)
  q_phase_voltage_per_switching_state4/1 -> MATLAB Function11/15(q_phase_voltage_per_switching_state)
  x_phase_voltage_per_switching_state5/1 -> MATLAB Function10/16(x_phase_voltage_per_switching_state)
  SampleTime_div_Lx15/1 -> MATLAB Function8/3(SampleTime_div_Lx), MATLAB Function9/3(SampleTime_div_Lx), MATLAB Function10/3(SampleTime_div_Lx), MATLAB Function11/3(SampleTime_div_Lx), MATLAB Function12/3(SampleTime_div_Lx), MATLAB Function13/3(SampleTime_div_Lx), MATLAB Function14/3(SampleTime_div_Lx), MATLAB Function15/3(SampleTime_div_Lx)
  SampleTime_div_Ly15/1 -> MATLAB Function8/4(SampleTime_div_Ly), MATLAB Function9/4(SampleTime_div_Ly), MATLAB Function10/4(SampleTime_div_Ly), MATLAB Function11/4(SampleTime_div_Ly), MATLAB Function12/4(SampleTime_div_Ly), MATLAB Function13/4(SampleTime_div_Ly), MATLAB Function14/4(SampleTime_div_Ly), MATLAB Function15/4(SampleTime_div_Ly)
  SampleTime_div_Lq15/1 -> MATLAB Function8/2(SampleTime_div_Lq), MATLAB Function9/2(SampleTime_div_Lq), MATLAB Function10/2(SampleTime_div_Lq), MATLAB Function11/2(SampleTime_div_Lq), MATLAB Function12/2(SampleTime_div_Lq), MATLAB Function13/2(SampleTime_div_Lq), MATLAB Function14/2(SampleTime_div_Lq), MATLAB Function15/2(SampleTime_div_Lq)
  x_phase_voltage_per_switching_state7/1 -> MATLAB Function8/16(x_phase_voltage_per_switching_state)
  q_phase_voltage_per_switching_state/1 -> MATLAB Function15/15(q_phase_voltage_per_switching_state)
  MATLAB Function15/1(J) -> J/1
  d_phase_voltage_per_switching_state5/1 -> MATLAB Function10/14(d_phase_voltage_per_switching_state)
  MATLAB Function10/1(J) -> J5/1
  y_phase_voltage_per_switching_state5/1 -> MATLAB Function10/17(y_phase_voltage_per_switching_state)
  q_phase_voltage_per_switching_state6/1 -> MATLAB Function9/15(q_phase_voltage_per_switching_state)
  y_phase_voltage_per_switching_state6/1 -> MATLAB Function9/17(y_phase_voltage_per_switching_state)
  x_phase_voltage_per_switching_state6/1 -> MATLAB Function9/16(x_phase_voltage_per_switching_state)
  MATLAB Function9/1(J) -> J6/1
  MATLAB Function12/1(J) -> J3/1
  q_phase_voltage_per_switching_state7/1 -> MATLAB Function8/15(q_phase_voltage_per_switching_state)
  y_phase_voltage_per_switching_state3/1 -> MATLAB Function12/17(y_phase_voltage_per_switching_state)
  q_phase_voltage_per_switching_state3/1 -> MATLAB Function12/15(q_phase_voltage_per_switching_state)
  ix_ref15/1 -> MATLAB Function8/20(ix_ref), MATLAB Function9/20(ix_ref), MATLAB Function10/20(ix_ref), MATLAB Function11/20(ix_ref), MATLAB Function12/20(ix_ref), MATLAB Function13/20(ix_ref), MATLAB Function14/20(ix_ref), MATLAB Function15/20(ix_ref)
  iq_ref15/1 -> MATLAB Function8/19(iq_ref), MATLAB Function9/19(iq_ref), MATLAB Function10/19(iq_ref), MATLAB Function11/19(iq_ref), MATLAB Function12/19(iq_ref), MATLAB Function13/19(iq_ref), MATLAB Function14/19(iq_ref), MATLAB Function15/19(iq_ref)
  id_ref15/1 -> MATLAB Function8/18(id_ref), MATLAB Function9/18(id_ref), MATLAB Function10/18(id_ref), MATLAB Function11/18(id_ref), MATLAB Function12/18(id_ref), MATLAB Function13/18(id_ref), MATLAB Function14/18(id_ref), MATLAB Function15/18(id_ref)
  Ld15/1 -> MATLAB Function8/12(Ld), MATLAB Function9/12(Ld), MATLAB Function10/12(Ld), MATLAB Function11/12(Ld), MATLAB Function12/12(Ld), MATLAB Function13/12(Ld), MATLAB Function14/12(Ld), MATLAB Function15/12(Ld)
  iy_k_16/1 -> MATLAB Function8/8(iy_k_1), MATLAB Function9/8(iy_k_1), MATLAB Function10/8(iy_k_1), MATLAB Function11/8(iy_k_1), MATLAB Function12/8(iy_k_1), MATLAB Function13/8(iy_k_1), MATLAB Function14/8(iy_k_1), MATLAB Function15/8(iy_k_1)
  ix_k_16/1 -> MATLAB Function8/7(ix_k_1), MATLAB Function9/7(ix_k_1), MATLAB Function10/7(ix_k_1), MATLAB Function11/7(ix_k_1), MATLAB Function12/7(ix_k_1), MATLAB Function13/7(ix_k_1), MATLAB Function14/7(ix_k_1), MATLAB Function15/7(ix_k_1)
  iq_k_16/1 -> MATLAB Function8/6(iq_k_1), MATLAB Function9/6(iq_k_1), MATLAB Function10/6(iq_k_1), MATLAB Function11/6(iq_k_1), MATLAB Function12/6(iq_k_1), MATLAB Function13/6(iq_k_1), MATLAB Function14/6(iq_k_1), MATLAB Function15/6(iq_k_1)
  id_k_16/1 -> MATLAB Function8/5(id_k_1), MATLAB Function9/5(id_k_1), MATLAB Function10/5(id_k_1), MATLAB Function11/5(id_k_1), MATLAB Function12/5(id_k_1), MATLAB Function13/5(id_k_1), MATLAB Function14/5(id_k_1), MATLAB Function15/5(id_k_1)

== matlab function FCS_MPC_6ph_testbench/Microcontroller Software/Switching_states/MATLAB Function1 ==
  data: I input; next_switching_state output
function next_switching_state = fcn(I)

    % Possible switching states of the 6-Phase 2-level inverter
    possible_swichting_states = [0	1	0	1	0	1	0	1	0	1	0	1;
                                1	0	0	1	0	1	0	1	0	1	0	1;
                                0	1	1	0	0	1	0	1	0	1	0	1;
                                1	0	1	0	0	1	0	1	0	1	0	1;
                                0	1	0	1	1	0	0	1	0	1	0	1;
                                1	0	0	1	1	0	0	1	0	1	0	1;
                                0	1	1	0	1	0	0	1	0	1	0	1;
                                1	0	1	0	1	0	0	1	0	1	0	1;
                                0	1	0	1	0	1	1	0	0	1	0	1;
                                1	0	0	1	0	1	1	0	0	1	0	1;
                                0	1	1	0	0	1	1	0	0	1	0	1;
                                1	0	1	0	0	1	1	0	0	1	0	1;
                                0	1	0	1	1	0	1	0	0	1	0	1;
                                1	0	0	1	1	0	1	0	0	1	0	1;
                                0	1	1	0	1	0	1	0	0	1	0	1;
                                1	0	1	0	1	0	1	0	0	1	0	1;
                                0	1	0	1	0	1	0	1	1	0	0	1;
                                1	0	0	1	0	1	0	1	1	0	0	1;
                                0	1	1	0	0	1	0	1	1	0	0	1;
                                1	0	1	0	0	1	0	1	1	0	0	1;
                                0	1	0	1	1	0	0	1	1	0	0	1;
                                1	0	0	1	1	0	0	1	1	0	0	1;
                                0	1	1	0	1	0	0	1	1	0	0	1;
                                1	0	1	0	1	0	0	1	1	0	0	1;
                                0	1	0	1	0	1	1	0	1	0	0	1;
                                1	0	0	1	0	1	1	0	1	0	0	1;
                                0	1	1	0	0	1	1	0	1	0	0	1;
                                1	0	1	0	0	1	1	0	1	0	0	1;
                                0	1	0	1	1	0	1	0	1	0	0	1;
                                1	0	0	1	1	0	1	0	1	0	0	1;
                                0	1	1	0	1	0	1	0	1	0	0	1;
                                1	0	1	0	1	0	1	0	1	0	0	1;
                                0	1	0	1	0	1	0	1	0	1	1	0;
                                1	0	0	1	0	1	0	1	0	1	1	0;
                                0	1	1	0	0	1	0	1	0	1	1	0;
                                1	0	1	0	0	1	0	1	0	1	1	0;
                                0	1	0	1	1	0	0	1	0	1	1	0;
                                1	0	0	1	1	0	0	1	0	1	1	0;
                                0	1	1	0	1	0	0	1	0	1	1	0;
                                1	0	1	0	1	0	0	1	0	1	1	0;
                                0	1	0	1	0	1	1	0	0	1	1	0;
                                1	0	0	1	0	1	1	0	0	1	1	0;
                                0	1	1	0	0	1	1	0	0	1	1	0;
                                1	0	1	0	0	1	1	0	0	1	1	0;
                                0	1	0	1	1	0	1	0	0	1	1	0;
                                1	0	0	1	1	0	1	0	0	1	1	0;
                                0	1	1	0	1	0	1	0	0	1	1	0;
                                1	0	1	0	1	0	1	0	0	1	1	0;
                                0	1	0	1	0	1	0	1	1	0	1	0;
                                1	0	0	1	0	1	0	1	1	0	1	0;
                                0	1	1	0	0	1	0	1	1	0	1	0;
                                1	0	1	0	0	1	0	1	1	0	1	0;
                                0	1	0	1	1	0	0	1	1	0	1	0;
                                1	0	0	1	1	0	0	1	1	0	1	0;
                                0	1	1	0	1	0	0	1	1	0	1	0;
                                1	0	1	0	1	0	0	1	1	0	1	0;
                                0	1	0	1	0	1	1	0	1	0	1	0;
                                1	0	0	1	0	1	1	0	1	0	1	0;
                                0	1	1	0	0	1	1	0	1	0	1	0;
                                1	0	1	0	0	1	1	0	1	0	1	0;
                                0	1	0	1	1	0	1	0	1	0	1	0;
                                1	0	0	1	1	0	1	0	1	0	1	0;
                                0	1	1	0	1	0	1	0	1	0	1	0;
                                1	0	1	0	1	0	1	0	1	0	1	0];

    % Initial condition
    if I==0
        I=int32(1);
    end

    % Output switching state
    next_switching_state=boolean(possible_swichting_states(I,:))';

end

== matlab function FCS_MPC_6ph_testbench/6ph_PMSM_30deg_VSD1 ==
  data: u1 input; y1 output; u2 input; u3 input; u4 input; u5 input; u6 input; y2 output; y3 output; y4 output; y5 output; y6 output; k6 input; c6 input
function [y1,y2,y3,y4,y5,y6] = VSD_asymm_30(u1,u2,u3,u4,u5,u6,k6,c6)

A =single([0 0 0 0 0 0]');

A =    k6*[1    -0.5        -0.5        sqrt(3)/2   -sqrt(3)/2  0 ;
           0    sqrt(3)/2   -sqrt(3)/2  0.5         0.5         -1;
           1    -0.5        -0.5        -sqrt(3)/2  sqrt(3)/2   0 ;
           0    -sqrt(3)/2  sqrt(3)/2   0.5         0.5         -1;
           c6   c6          c6          0           0           0 ;
           0    0           0           c6          c6          c6] * [u1 u2 u3 u4 u5 u6]';

y1 =single(A(1));
y2 =single(A(2));
y3 =single(A(3));
y4 =single(A(4));
y5 =single(A(5));
y6 =single(A(6));

== matlab function FCS_MPC_6ph_testbench/Microcontroller Software/Prediction_and_cost_function/Subsystem/MATLAB Function8 ==
  data: SampleTime_div_Ld input; J output; SampleTime_div_Lq input; SampleTime_div_Lx input; SampleTime_div_Ly input; id_k_1 input; iq_k_1 input; ix_k_1 input; iy_k_1 input; Rs input; omega_el input; Lq input; Ld input; psiPM input; d_phase_voltage_per_switching_state input; q_phase_voltage_per_switching_state input; x_phase_voltage_per_switching_state input; y_phase_voltage_per_switching_state input; id_ref input; iq_ref input; ix_ref input; iy_ref input
function J = fcn(SampleTime_div_Ld, SampleTime_div_Lq, SampleTime_div_Lx, SampleTime_div_Ly, id_k_1, iq_k_1, ix_k_1, iy_k_1, Rs, omega_el, Lq, Ld, psiPM, d_phase_voltage_per_switching_state, q_phase_voltage_per_switching_state, x_phase_voltage_per_switching_state, y_phase_voltage_per_switching_state, id_ref, iq_ref, ix_ref, iy_ref)
     
        % Prediction of the d-, q-, x-, y-currents of the 6-Phase-PMSM with the finite control set 
        id_k_2 = single(SampleTime_div_Ld*(d_phase_voltage_per_switching_state-id_k_1*Rs+omega_el*Lq*iq_k_1)+id_k_1);
        iq_k_2 = single(SampleTime_div_Lq*(q_phase_voltage_per_switching_state-iq_k_1*Rs-omega_el*(psiPM+id_k_1*Ld))+iq_k_1);
        ix_k_2 = single(SampleTime_div_Lx*(x_phase_voltage_per_switching_state-ix_k_1*Rs)+ix_k_1);
        iy_k_2 = single(SampleTime_div_Ly*(y_phase_voltage_per_switching_state-iy_k_1*Rs)+iy_k_1);
        
        % Calculation of the cost function
        J = single((id_ref-id_k_2)^2+(iq_ref-iq_k_2)^2+(ix_ref-ix_k_2)^2+(iy_ref-iy_k_2)^2);

end

== matlab function FCS_MPC_6ph_testbench/Microcontroller Software/Prediction_and_cost_function/Subsystem/MATLAB Function9 ==
  data: SampleTime_div_Ld input; J output; SampleTime_div_Lq input; SampleTime_div_Lx input; SampleTime_div_Ly input; id_k_1 input; iq_k_1 input; ix_k_1 input; iy_k_1 input; Rs input; omega_el input; Lq input; Ld input; psiPM input; d_phase_voltage_per_switching_state input; q_phase_voltage_per_switching_state input; x_phase_voltage_per_switching_state input; y_phase_voltage_per_switching_state input; id_ref input; iq_ref input; ix_ref input; iy_ref input
function J = fcn(SampleTime_div_Ld, SampleTime_div_Lq, SampleTime_div_Lx, SampleTime_div_Ly, id_k_1, iq_k_1, ix_k_1, iy_k_1, Rs, omega_el, Lq, Ld, psiPM, d_phase_voltage_per_switching_state, q_phase_voltage_per_switching_state, x_phase_voltage_per_switching_state, y_phase_voltage_per_switching_state, id_ref, iq_ref, ix_ref, iy_ref)
     
        % Prediction of the d-, q-, x-, y-currents of the 6-Phase-PMSM with the finite control set 
        id_k_2 = single(SampleTime_div_Ld*(d_phase_voltage_per_switching_state-id_k_1*Rs+omega_el*Lq*iq_k_1)+id_k_1);
        iq_k_2 = single(SampleTime_div_Lq*(q_phase_voltage_per_switching_state-iq_k_1*Rs-omega_el*(psiPM+id_k_1*Ld))+iq_k_1);
        ix_k_2 = single(SampleTime_div_Lx*(x_phase_voltage_per_switching_state-ix_k_1*Rs)+ix_k_1);
        iy_k_2 = single(SampleTime_div_Ly*(y_phase_voltage_per_switching_state-iy_k_1*Rs)+iy_k_1);
        
        % Calculation of the cost function
        J = single((id_ref-id_k_2)^2+(iq_ref-iq_k_2)^2+(ix_ref-ix_k_2)^2+(iy_ref-iy_k_2)^2);

end
